simulink model "Exemplo_Robo1dof"  (R2015a)
settings: Solver=ode5  StartTime=0.0  StopTime=1000  FixedStep=0.01  MaxStep=1  RelTol=1e-3
libraries: simulink x3, AvgModels x1
settings Model: CovSFcnEnable=off  Creator=lgalotto  LastModifiedBy=lgalo
settings DataIOCC: SignalLoggingSaveFormat=ModelDataLogs
settings OptimizationCC: ExpressionDepthLimit=2147483647
settings DebuggingCC: UnderspecifiedInitializationDetection=Classic  MergeDetectMultiDrivingBlocksExec=none  SolverPrmCheckMsg=warning  FcnCallInpInsideContextMsg=EnableAllAsWarning  StateNameClashWarn=warning
settings GRTTargetCC: CombineOutputUpdateFcns=off  GRTInterface=on

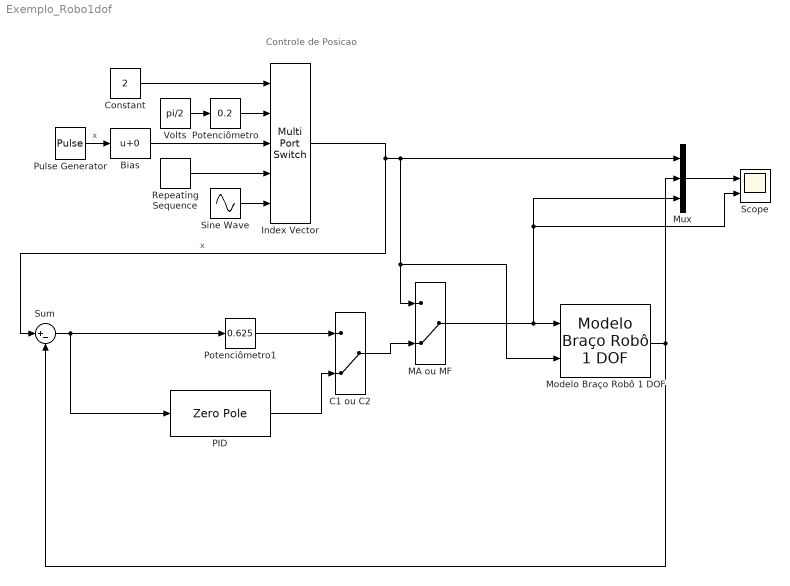
== system Exemplo_Robo1dof ==
  note: Controle de Posicao
  Bias : Bias
  C1 ou C2 : ManualSwitch  CurrentSetting=0
  Constant : Constant  Value=2
  Index Vector : MultiPortSwitch  DataPortOrder=Zero-based contiguous  Inputs=4  zeroidx=on
  MA ou MF : ManualSwitch  CurrentSetting=0
  Modelo Braço Robô 1 DOF : AvgModels/Modelos Animados/Modelo Braço Robô 1 DOF  J=1  K=0.1
  Mux : Mux  Inputs=3
  PID : ZeroPole  Zeros=[-0.2 -0.2]  Poles=[0 -2]  Gain=[55.5]
  Potenciômetro : simulink/Math Operations/Slider Gain  low=-1  gain=0.2  high=1
  Potenciômetro1 : simulink/Math Operations/Slider Gain  low=0  gain=0.625  high=0.625
  Pulse Generator : DiscretePulseGenerator  PulseType=Time based  Amplitude=pi/2  Period=100  PulseWidth=50
  Repeating Sequence : simulink/Sources/Repeating Sequence  rep_seq_t=[0 60 120]  rep_seq_y=[0 4*pi 0]
  Scope : Scope  NumInputPorts=2
      settings: YMin=-5~-5  YMax=5~5
  Sine Wave : Sin  Frequency=0.2  SampleTime=0
  Sum : Sum  Inputs=|+-
  Volts : Constant  Value=pi/2
  wires:
  Index Vector/1 -> Mux/1, Modelo Braço Robô 1 DOF/2, MA ou MF/1, Sum/1  "x"
  Mux/1 -> Scope/1
  Pulse Generator/1 -> Bias/1  "x"
  Constant/1 -> Index Vector/1
  Sine Wave/1 -> Index Vector/5
  Modelo Braço Robô 1 DOF/1 -> Mux/2, Sum/2
  Repeating Sequence/1 -> Index Vector/4
  MA ou MF/1 -> Modelo Braço Robô 1 DOF/1, Mux/3, Scope/2
  Bias/1 -> Index Vector/3
  Volts/1 -> Potenciômetro/1
  Potenciômetro/1 -> Index Vector/2
  PID/1 -> C1 ou C2/2
  C1 ou C2/1 -> MA ou MF/2
  Sum/1 -> Potenciômetro1/1, PID/1
  Potenciômetro1/1 -> C1 ou C2/1
